simulink subsystem "Model_LAB4_controller_robusttrack"  (R2024b)
settings: Solver=VariableStepAuto  StartTime=0.0  StopTime=10.0  RelTol=1e-3
values from neighbouring files (symbols this model uses):
  Nu = Sol(5,:)    [A_final_results.m]
  Nx = Sol(1:4,:)    [A_final_results.m]
undefined symbols (not defined in the file or in its folder): DiscIntNeverNeededParam, K_fb, Ki, V2duty
settings Model: Creator=Utente  LastModifiedBy=Utente

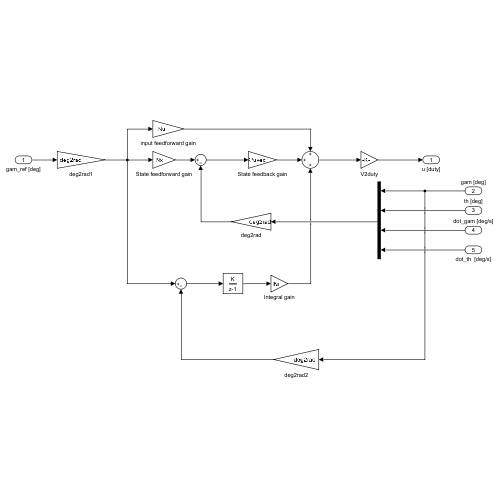
[thumbnail: Simulink's stored preview of the top-level diagram]
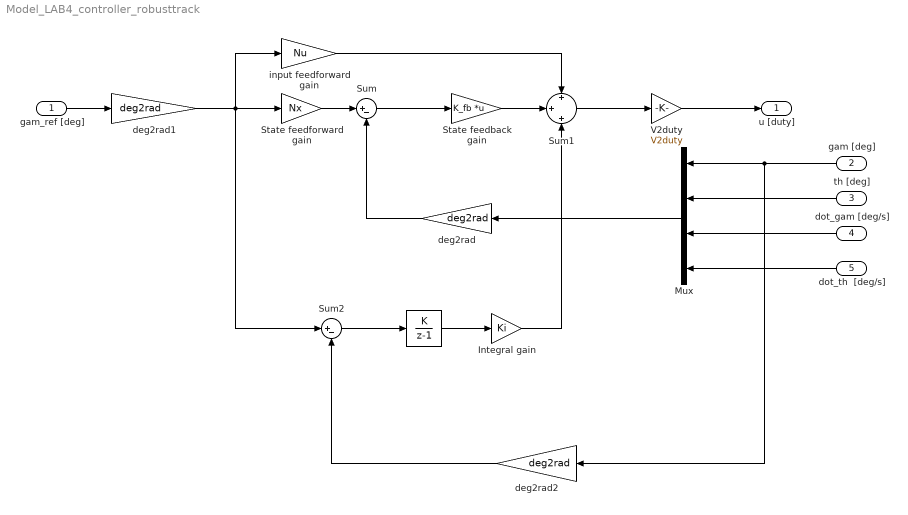
== system Model_LAB4_controller_robusttrack ==
  gam_ref [deg] : Inport
  gam [deg] : Inport  Port=2
  th [deg] : Inport  Port=3
  dot_gam [deg/s] : Inport  Port=4
  dot_th  [deg/s] : Inport  Port=5
  " " : DiscreteIntegrator  IntegratorMethod=Accumulation: Forward Euler  SampleTime=-1  ICPrevOutput=DiscIntNeverNeededParam  ICPrevScaledInput=DiscIntNeverNeededParam
  Integral gain : Gain  Gain=Ki
  Mux : Mux
  State feedback gain : Gain  Gain=K_fb  Multiplication=Matrix(K*u) (u vector)
  State feedforward gain : Gain  Gain=Nx
  Sum : Sum  Inputs=|+-
  Sum1 : Sum  Inputs=+|+|+
  Sum2 : Sum  Inputs=|+-
  V2duty : Gain  Gain=V2duty
  deg2rad : Gain  Gain=deg2rad
  deg2rad1 : Gain  Gain=deg2rad
  deg2rad2 : Gain  Gain=deg2rad
  input feedforward gain : Gain  Gain=Nu
  u [duty] : Outport
  wires:
  Sum1/1 -> V2duty/1
  V2duty/1 -> u [duty]/1
  deg2rad/1 -> Sum/2
  gam [deg]/1 -> deg2rad2/1, Mux/1
  dot_th  [deg/s]/1 -> Mux/4
  dot_gam [deg/s]/1 -> Mux/3
  Mux/1 -> deg2rad/1
  th [deg]/1 -> Mux/2
  input feedforward gain/1 -> Sum1/1
  deg2rad1/1 -> Sum2/1, input feedforward gain/1, State feedforward gain/1
  Sum/1 -> State feedback gain/1
  gam_ref [deg]/1 -> deg2rad1/1
  State feedforward gain/1 -> Sum/1
  State feedback gain/1 -> Sum1/2
  deg2rad2/1 -> Sum2/2
  Sum2/1 -> " "/1
  " "/1 -> Integral gain/1
  Integral gain/1 -> Sum1/3
